simulink model "volo_agcdc_pipelined"  (R2012b)
settings: Solver=ode45  StartTime=0.0  StopTime=1000  RelTol=1e-3
PreLoadFcn:
  | volo_agcdc_init
InitFcn:
  | volo_agcdc_init
StartFcn:
  | volo_agcdc_init
values from neighbouring files (symbols this model uses):
  agc_idleState = 0    [volo_agcdc_init.m]
  agc_numAddrBits = agc_numOutputs + agc_numStateBits    [volo_agcdc_init.m]
  regDCRemoval_AvgLength = 64    [volo_agcdc_init.m]
  regSatDet_NumSamples = 16    [volo_agcdc_init.m]
undefined symbols (not defined in the file or in its folder): gcbh, xlBlockLoadCallback, xlGetNormalizedPeriod
libraries: xbsIndex_r4 x681, xbsEDKLib_r4 x1
(part 6 of 7)

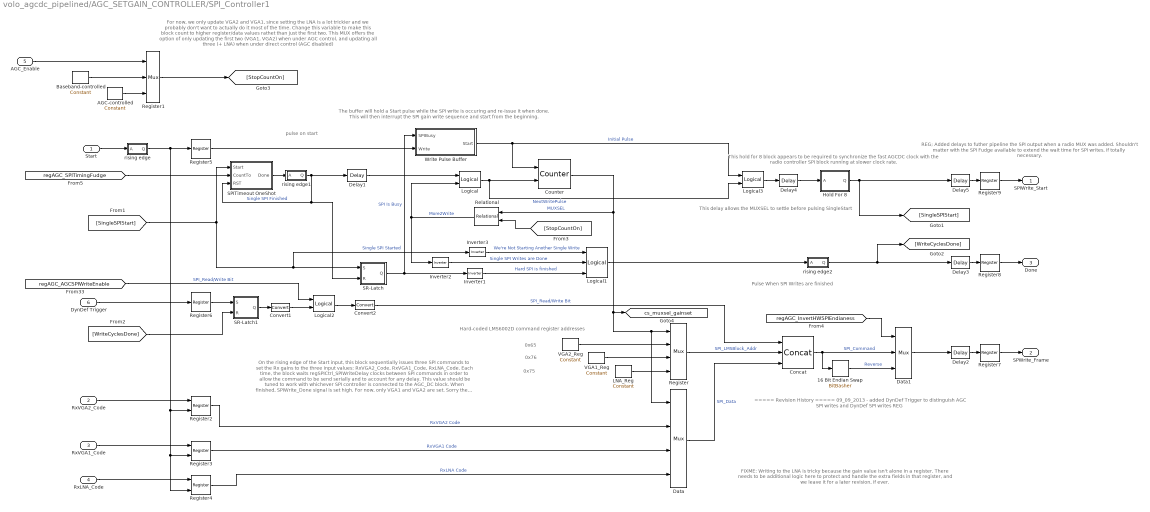
== system volo_agcdc_pipelined/AGC_SETGAIN_CONTROLLER/SPI_Controller1 ==
  note: REG; Added delays to futher pipeline the SPI output when a radio MUX was added.
      | Shouldn't matter with the SPI Fudge available to extend the wait time for SPI writes,
      | if totally necessary.
  note: This hold for 8 block appears to be required
      | to synchronize the fast AGCDC clock with
      | the radio controller SPI block running at slower
      | clock rate.
  note: ===== Revision History =====
      | 09_09_2013 - added DynDef Trigger to distinguish AGC SPI writes and DynDef SPI writes REG
  note: FIXME: Writing to the LNA is tricky because the gain value isn't alone in a register. There needs
      | to be additional logic here to protect and handle the extra fields in that register, and we leave it
      | for a later revision, if ever.
  note: For now, we only update VGA2 and VGA1, since setting the LNA is a lot trickier and we
      | probably don't want to actually do it most of the time. Change this variable to make this
      | block count to higher register/data values rathet than just the first two. This MUX offers the
      | option of only updating the first two (VGA1, VGA2) when under AGC control, and updating all
      | three (+ LNA) when under direct control (AGC disabled)
  note: The buffer will hold a Start pulse while the SPI write is occuring and re-issue it when done.
      | This will then interrupt the SPI gain write sequence and start from the beginning.
  note: This delay allows the MUXSEL
      | to settle before pulsing SingleStart
  note: Pulse When SPI Writes are finished
  note: pulse on start
  note: 0x75
  note: 0x76
  note: 0x65
  note: Hard-coded LMS6002D command
      | register addresses
  note: On the rising edge of the Start input, this block sequentially issues three SPI commands
      | to set the Rx gains to the three input values: RxVGA2_Code, RxVGA1_Code, RxLNA_Code.
      | Each time, the block waits regSPICtrl_SPIWriteDelay clocks between SPI commands in order
      | to allow the command to be send serially and to account for any delay. This value should be tuned
      | to work with whichever SPI controller is connected to the AGC_DC block. When finished,
      | SPIWrite_Done signal is set high. For now, only VGA1 and VGA2 are set.
      | Sorry the logic is a cluster, that's my bad--we had some serious issues with the SPI controller block.
      | me@ryaneguerra.com
      | June 15, 2013
  Start : Inport
  RxVGA2_Code : Inport  Port=2
  RxVGA1_Code : Inport  Port=3
  RxLNA_Code : Inport  Port=4
  AGC_Enable : Inport  Port=5
  DynDef Trigger : Inport  Port=6
  16 Bit Endian Swap : xbsIndex_r4/BitBasher  bitexpr=|  display_expr=off  sr_1=1  arith_type1=Unsigned  bin_pt1=0  sr_2=2  arith_type2=Unsigned  bin_pt2=0  sr_3=3  arith_type3=Unsigned  bin_pt3=0  sr_4=4  arith_type4=Unsigned  bin_pt4=0  dbl_ovrd=off  block_type=bitbasher
      | <!DOCTYPE HTML PUBLIC "-//W3C//DTD HTML 4.0//EN" "http://www.w3.org/TR/REC-html40/strict.dtd">
      | <html><head><meta name="qrichtext" content="1" /><style type="text/css">
      | p, li { white-space: pre-wrap; }
      | </style></head><body style=" font-family:'MS Shell Dlg 2'; font-size:8.25pt; font-weight:400; font-style:normal;">
      | <p style=" margin-top:12px; margin-bottom:12px; margin-left:0px; margin-right:0px; -qt-block-indent:0; text-indent:0px;"><span style=" font-family:'MS Shell Dlg'; font-size:8pt;">a={b[0:15]}</span></p></body></html>
  AGC-controlled : xbsIndex_r4/Constant  const=1  gui_display_data_type=Fixed-point  arith_type=Unsigned  n_bits=2  bin_pt=0  preci_type=Single  exp_width=8  frac_width=24  explicit_period=off  period=1  equ=P=C  opselect=C  inp2=PCIN>>17  opr=+  inp1=P  carry=CIN  dbl_ovrd=off  block_type=constant
  Baseband-controlled : xbsIndex_r4/Constant  const=1  gui_display_data_type=Fixed-point  arith_type=Unsigned  n_bits=2  bin_pt=0  preci_type=Single  exp_width=8  frac_width=24  explicit_period=off  period=1  equ=P=C  opselect=C  inp2=PCIN>>17  opr=+  inp1=P  carry=CIN  dbl_ovrd=off  block_type=constant
  Concat : xbsIndex_r4/Concat  num_inputs=3  dbl_ovrd=off  block_type=concat
  Convert1 : xbsIndex_r4/Convert  gui_display_data_type=Boolean  arith_type=Boolean  n_bits=16  bin_pt=14  float_type=Single  exp_bits=8  fraction_bits=24  quantization=Truncate  overflow=Wrap  en=off  latency=0  dbl_ovrd=off  pipeline=off  block_type=convert
  Convert2 : xbsIndex_r4/Convert  gui_display_data_type=Fixed-point  arith_type=Unsigned  n_bits=1  bin_pt=0  float_type=Single  exp_bits=8  fraction_bits=24  quantization=Truncate  overflow=Wrap  en=off  latency=0  dbl_ovrd=off  pipeline=off  block_type=convert
  Counter : xbsIndex_r4/Counter  cnt_type=Free Running  cnt_to=Inf  operation=Up  start_count=0  cnt_by_val=1  arith_type=Unsigned  n_bits=2  bin_pt=0  load_pin=off  rst=on  en=on  explicit_period=on  period=1  dbl_ovrd=off  use_behavioral_HDL=off  implementation=Fabric  block_type=counter
  Data : xbsIndex_r4/Mux  inputs=3  en=off  latency=0  precision=Full  arith_type=Unsigned  n_bits=16  bin_pt=14  quantization=Truncate  overflow=Wrap  dbl_ovrd=off  block_type=mux
  Data1 : xbsIndex_r4/Mux  inputs=2  en=off  latency=0  precision=Full  arith_type=Unsigned  n_bits=16  bin_pt=14  quantization=Truncate  overflow=Wrap  dbl_ovrd=off  block_type=mux
  Delay{1..5} (5 alike) : xbsIndex_r4/Delay  rst=off  infoeditControl=Selection of Reset will increase slice count due to use of real FFs and instead of SRLs  en=off  latency=1  dbl_ovrd=off  reg_retiming=off  block_type=delay
  Hold For 8 : Subsystem
  Inverter1 : xbsIndex_r4/Inverter  en=off  latency=0  dbl_ovrd=off  block_type=inv
  Inverter2 : xbsIndex_r4/Inverter  en=off  latency=0  dbl_ovrd=off  block_type=inv
  Inverter3 : xbsIndex_r4/Inverter  en=off  latency=0  dbl_ovrd=off  block_type=inv
  LNA_Reg : xbsIndex_r4/Constant  const=hex2dec('75')  gui_display_data_type=Fixed-point  arith_type=Unsigned  n_bits=7  bin_pt=0  preci_type=Single  exp_width=8  frac_width=24  explicit_period=on  period=1  equ=P=C  opselect=C  inp2=PCIN>>17  opr=+  inp1=P  carry=CIN  dbl_ovrd=off  block_type=constant
  Logical : xbsIndex_r4/Logical  logical_function=AND  inputs=2  en=off  latency=0  precision=Full  arith_type=Unsigned  n_bits=16  bin_pt=0  align_bp=on  dbl_ovrd=off  block_type=logical
  Logical1 : xbsIndex_r4/Logical  logical_function=AND  inputs=3  en=off  latency=0  precision=Full  arith_type=Unsigned  n_bits=16  bin_pt=0  align_bp=on  dbl_ovrd=off  block_type=logical
  Logical2 : xbsIndex_r4/Logical  logical_function=OR  inputs=2  en=off  latency=0  precision=Full  arith_type=Unsigned  n_bits=16  bin_pt=0  align_bp=on  dbl_ovrd=off  block_type=logical
  Logical3 : xbsIndex_r4/Logical  logical_function=OR  inputs=2  en=off  latency=0  precision=Full  arith_type=Unsigned  n_bits=16  bin_pt=0  align_bp=on  dbl_ovrd=off  block_type=logical
  Register : xbsIndex_r4/Mux  inputs=3  en=off  latency=0  precision=Full  arith_type=Unsigned  n_bits=16  bin_pt=14  quantization=Truncate  overflow=Wrap  dbl_ovrd=off  block_type=mux
  Register1 : xbsIndex_r4/Mux  inputs=2  en=off  latency=0  precision=Full  arith_type=Unsigned  n_bits=16  bin_pt=14  quantization=Truncate  overflow=Wrap  dbl_ovrd=off  block_type=mux
  Register2 : xbsIndex_r4/Register  init=0  rst=off  en=on  dbl_ovrd=off  block_type=register
  Register3 : xbsIndex_r4/Register  init=0  rst=off  en=on  dbl_ovrd=off  block_type=register
  Register4 : xbsIndex_r4/Register  init=0  rst=off  en=on  dbl_ovrd=off  block_type=register
  Register{5..9} (5 alike) : xbsIndex_r4/Register  init=0  rst=off  en=off  dbl_ovrd=off  block_type=register
  Relational : xbsIndex_r4/Relational  mode=a<b  en=off  latency=0  dbl_ovrd=off  block_type=relational
  SPITimeout OneShot : Subsystem
  SR-Latch : Subsystem
  SR-Latch1 : Subsystem
  VGA1_Reg : xbsIndex_r4/Constant  const=hex2dec('76')  gui_display_data_type=Fixed-point  arith_type=Unsigned  n_bits=7  bin_pt=0  preci_type=Single  exp_width=8  frac_width=24  explicit_period=on  period=1  equ=P=C  opselect=C  inp2=PCIN>>17  opr=+  inp1=P  carry=CIN  dbl_ovrd=off  block_type=constant
  VGA2_Reg : xbsIndex_r4/Constant  const=hex2dec('65')  gui_display_data_type=Fixed-point  arith_type=Unsigned  n_bits=7  bin_pt=0  preci_type=Single  exp_width=8  frac_width=24  explicit_period=on  period=1  equ=P=C  opselect=C  inp2=PCIN>>17  opr=+  inp1=P  carry=CIN  dbl_ovrd=off  block_type=constant
  Write Pulse Buffer : Subsystem
  rising edge : Subsystem
  rising edge1 : Subsystem
  rising edge2 : Subsystem
  SPIWrite_Start : Outport
  SPWrite_Frame : Outport  Port=2
  Done : Outport  Port=3
  tag scope: cs_muxsel_gainset=global
  wires:
  Register3/1 -> Data/3  "RxVGA1 Code"
  Register4/1 -> Data/4  "RxLNA Code"
  Register2/1 -> Data/2  "RxVGA2 Code"
  VGA1_Reg/1 -> Register/3
  LNA_Reg/1 -> Register/4
  VGA2_Reg/1 -> Register/2
  Data/1 -> Concat/3  "SPI_Data"
  Register/1 -> Concat/2  "SPI_LMSBlock_Addr"
  Concat/1 -> Data1/2, 16 Bit Endian Swap/1  "SPI_Command"
  Counter/1 -> Data/1, Register/1, [cs_muxsel_gainset], Relational/1  "MUXSEL"
  [StopCountOn] -> Relational/2
  Logical1/1 -> rising edge2/1(A)
  Register1/1 -> [StopCountOn]
  Logical2/1 -> Convert2/1
  SR-Latch/1(Q) -> Inverter1/1, Write Pulse Buffer/1(SPIBusy)  "SPI Is Busy"
  Relational/1 -> Inverter2/1, Logical/2  "More2Write"
  rising edge1/1(Q) -> SPITimeout OneShot/3(RST), SR-Latch/2(R), Delay1/1  "Single SPI Finished"
  Inverter2/1 -> Logical1/2  "Single SPI Writes are Done"
  Start/1 -> rising edge/1(A)
  Register5/1 -> Write Pulse Buffer/2(Write)
  Write Pulse Buffer/1(Start) -> Logical3/1, Counter/1  "Initial Pulse"
  rising edge2/1(Q) -> Delay3/1, [WriteCyclesDone]
  [SingleSPIStart] -> SR-Latch/1(S), Inverter3/1, SPITimeout OneShot/1(Start)  "Single SPI Started"
  Inverter1/1 -> Logical1/3  "Hard SPI is finished"
  [regAGC_SPITimingFudge] -> SPITimeout OneShot/2(CountTo)
  SPITimeout OneShot/1(Done) -> rising edge1/1(A)
  Delay1/1 -> Logical/1
  Logical/1 -> Logical3/2, Counter/2  "NextWritePulse"
  Inverter3/1 -> Logical1/1  "We're Not Starting Another Single Write"
  AGC-controlled/1 -> Register1/3
  Baseband-controlled/1 -> Register1/2
  AGC_Enable/1 -> Register1/1
  [regAGC_AGCSPIWriteEnable] -> Logical2/1  "SPI_Read/Write Bit"
  DynDef Trigger/1 -> Register6/1
  SR-Latch1/1(Q) -> Convert1/1
  [WriteCyclesDone] -> SR-Latch1/2(R)
  Convert1/1 -> Logical2/2
  Convert2/1 -> Concat/1  "SPI_Read/Write Bit"
  [regAGC_InvertHWSPIEndianess] -> Data1/1
  16 Bit Endian Swap/1 -> Data1/3  "Reverse"
  Data1/1 -> Delay2/1
  RxLNA_Code/1 -> Register4/1
  RxVGA1_Code/1 -> Register3/1
  RxVGA2_Code/1 -> Register2/1
  rising edge/1(Q) -> Register4/2, Register3/2, Register2/2, Register5/1
  Register6/1 -> SR-Latch1/1(S)
  Hold For 8/1(Q) -> Delay5/1, [SingleSPIStart]
  Logical3/1 -> Delay4/1
  Delay4/1 -> Hold For 8/1(A)
  Register7/1 -> SPWrite_Frame/1
  Delay2/1 -> Register7/1
  Delay3/1 -> Register8/1
  Register8/1 -> Done/1
  Register9/1 -> SPIWrite_Start/1
  Delay5/1 -> Register9/1

== system volo_agcdc_pipelined/AGC_SETGAIN_CONTROLLER/SR-Latch ==
  S : Inport
  R : Inport  Port=2
  Register : xbsIndex_r4/Register  init=0  rst=on  en=on  dbl_ovrd=off  block_type=register
  Q : Outport
  wires:
  S/1 -> Register/3, Register/1
  Register/1 -> Q/1
  R/1 -> Register/2

== system volo_agcdc_pipelined/AGC_SETGAIN_CONTROLLER/rising edge ==
  note: rising edge
  A : Inport
  Delay1 : xbsIndex_r4/Delay  rst=off  infoeditControl=Selection of Reset will increase slice count due to use of real FFs and instead of SRLs  en=off  latency=1  dbl_ovrd=off  reg_retiming=off  block_type=delay
  Inverter2 : xbsIndex_r4/Inverter  en=off  latency=0  dbl_ovrd=off  block_type=inv
  Logical2 : xbsIndex_r4/Logical  logical_function=AND  inputs=2  en=off  latency=0  precision=Full  arith_type=Unsigned  n_bits=16  bin_pt=0  align_bp=on  dbl_ovrd=off  block_type=logical
  Q : Outport
  wires:
  Logical2/1 -> Q/1
  A/1 -> Logical2/1, Delay1/1
  Delay1/1 -> Inverter2/1
  Inverter2/1 -> Logical2/2

== system volo_agcdc_pipelined/DC_REMOVAL/Sliding Sum 64_1 ==
  in : Inport
  rst : Inport  Port=2
  RxValid : Inport  Port=3
  Accum1 : xbsIndex_r4/Accumulator  operation=Add  n_bits=22  overflow=Saturate  scale=1  rst=on  infoeditControl=reset for floating point data type must be asserted for a minimum of 2 cycles  hasbypass=off  en=on  latency=0  dbl_ovrd=off  msb_inp=100  msb=100  lsb=-100  use_behavioral_HDL=on  implementation=Fabric  block_type=accum
      settings: xl_area=[12 23 0 22 0 0 0]  block_version=VER_STRING_GOES_HERE
  AddSub1 : xbsIndex_r4/AddSub  mode=Subtraction  use_carryin=off  use_carryout=off  en=off  latency=0  precision=Full  arith_type="Signed  (2's comp)"  n_bits=36  bin_pt=28  quantization=Truncate  overflow=Saturate  dbl_ovrd=off  use_behavioral_HDL=on  hw_selection=Fabric  pipelined=off  use_rpm=off  block_type=addsub
      settings: xl_area=[9 18 0 17 0 0 0]  block_version=VER_STRING_GOES_HERE
  Delay : xbsIndex_r4/Delay  rst=on  infoeditControl=Selection of Reset will increase slice count due to use of real FFs and instead of SRLs  en=on  latency=64  dbl_ovrd=off  reg_retiming=off  block_type=delay
  Out : Outport
  wires:
  Accum1/1 -> Out/1  "Sum"
  in/1 -> Delay/1, AddSub1/1  "Instantaneous"
  AddSub1/1 -> Accum1/1
  rst/1 -> Delay/2, Accum1/2
  Delay/1 -> AddSub1/2
  RxValid/1 -> Accum1/3, Delay/3

== system volo_agcdc_pipelined/DC_REMOVAL/Sliding Sum 64_2 ==
  in : Inport
  rst : Inport  Port=2
  RxValid : Inport  Port=3
  Accum1 : xbsIndex_r4/Accumulator  operation=Add  n_bits=22  overflow=Saturate  scale=1  rst=on  infoeditControl=reset for floating point data type must be asserted for a minimum of 2 cycles  hasbypass=off  en=on  latency=0  dbl_ovrd=off  msb_inp=100  msb=100  lsb=-100  use_behavioral_HDL=on  implementation=Fabric  block_type=accum
      settings: xl_area=[12 23 0 22 0 0 0]  block_version=VER_STRING_GOES_HERE
  AddSub1 : xbsIndex_r4/AddSub  mode=Subtraction  use_carryin=off  use_carryout=off  en=off  latency=0  precision=Full  arith_type="Signed  (2's comp)"  n_bits=36  bin_pt=28  quantization=Truncate  overflow=Saturate  dbl_ovrd=off  use_behavioral_HDL=on  hw_selection=Fabric  pipelined=off  use_rpm=off  block_type=addsub
      settings: xl_area=[9 18 0 17 0 0 0]  block_version=VER_STRING_GOES_HERE
  Delay : xbsIndex_r4/Delay  rst=on  infoeditControl=Selection of Reset will increase slice count due to use of real FFs and instead of SRLs  en=on  latency=64  dbl_ovrd=off  reg_retiming=off  block_type=delay
  Out : Outport
  wires:
  Accum1/1 -> Out/1  "Sum"
  in/1 -> Delay/1, AddSub1/1  "Instantaneous"
  AddSub1/1 -> Accum1/1
  rst/1 -> Delay/2, Accum1/2
  Delay/1 -> AddSub1/2
  RxValid/1 -> Delay/3, Accum1/3

== system volo_agcdc_pipelined/DC_REMOVAL/Valid Avg Counter ==
  RxValid : Inport
  RST : Inport  Port=2
  Constant : xbsIndex_r4/Constant  const=64  gui_display_data_type=Fixed-point  arith_type=Unsigned  n_bits=7  bin_pt=0  preci_type=Single  exp_width=8  frac_width=24  explicit_period=on  period=1  equ=P=C  opselect=C  inp2=PCIN>>17  opr=+  inp1=P  carry=CIN  dbl_ovrd=off  block_type=constant
  Counter : xbsIndex_r4/Counter  cnt_type=Free Running  cnt_to=10  operation=Up  start_count=0  cnt_by_val=1  arith_type=Unsigned  n_bits=ceil(log(regDCRemoval_AvgLength)/log(2))+1  bin_pt=0  load_pin=off  rst=on  en=on  explicit_period=on  period=1  dbl_ovrd=off  use_behavioral_HDL=off  implementation=Fabric  block_type=counter
  Inverter : xbsIndex_r4/Inverter  en=off  latency=0  dbl_ovrd=off  block_type=inv
  Logical : xbsIndex_r4/Logical  logical_function=AND  inputs=2  en=off  latency=0  precision=Full  arith_type=Unsigned  n_bits=16  bin_pt=0  align_bp=on  dbl_ovrd=off  block_type=logical
  Relational4 : xbsIndex_r4/Relational  mode=a>b  en=off  latency=0  dbl_ovrd=off  block_type=relational
  DCMeas_Good : Outport
  wires:
  RxValid/1 -> Logical/1
  RST/1 -> Counter/1
  Relational4/1 -> DCMeas_Good/1, Inverter/1  "DCMeasure_Good"
  Counter/1 -> Relational4/1
  Constant/1 -> Relational4/2
  Inverter/1 -> Logical/2  "keep_counting"
  Logical/1 -> Counter/2

== system volo_agcdc_pipelined/DynamicNoiseFloorAdjustment/Bounds Checking ==
  note: Note, it is not expected that the input is both above the max and below the min;
      | this is undefined behavior. Just to make sure nothing stupid happened, we'll put the
      | gain at MAX if that happens.
  note: Checks for rational bounds on the Dyn Default Gain,
      | otherwise, the output value is the rail value.
  NextGain_In : Inport
  Concat : xbsIndex_r4/Concat  num_inputs=2  dbl_ovrd=off  block_type=concat
  Delay1 : xbsIndex_r4/Delay  rst=off  infoeditControl=Selection of Reset will increase slice count due to use of real FFs and instead of SRLs  en=off  latency=1  dbl_ovrd=off  reg_retiming=off  block_type=delay
  Delay5 : xbsIndex_r4/Delay  rst=off  infoeditControl=Selection of Reset will increase slice count due to use of real FFs and instead of SRLs  en=off  latency=1  dbl_ovrd=off  reg_retiming=off  block_type=delay
  Mux : xbsIndex_r4/Mux  inputs=4  en=off  latency=0  precision=Full  arith_type=Unsigned  n_bits=16  bin_pt=14  quantization=Truncate  overflow=Wrap  dbl_ovrd=off  block_type=mux
  Relational : xbsIndex_r4/Relational  mode=a>b  en=off  latency=0  dbl_ovrd=off  block_type=relational
  Relational1 : xbsIndex_r4/Relational  mode=a<b  en=off  latency=0  dbl_ovrd=off  block_type=relational
  NextGain_Out : Outport
  wires:
  [regAGC_DynAdjustment_MinDefaultGain] -> Mux/4, Relational1/2  "Min Default Gain"
  [regAGC_DynAdjustment_MaxDefaultGain] -> Mux/5, Mux/3, Relational/2  "Max Default Gain"
  NextGain_In/1 -> Relational1/1, Relational/1, Delay1/1  "NExt Gain"
  Relational1/1 -> Concat/1  "IN < MIN"
  Relational/1 -> Concat/2  "IN > MAX"
  Concat/1 -> Delay5/1
  Delay5/1 -> Mux/1
  Delay1/1 -> Mux/2  "Next Gain"
  Mux/1 -> NextGain_Out/1

== system volo_agcdc_pipelined/DynamicNoiseFloorAdjustment/Default Gain Change Holdoff Timer ==
  Current_Default : Inport
  Next_Default : Inport  Port=2
  RST : Inport  Port=3
  Always Update : xbsIndex_r4/Constant  const=1  gui_display_data_type=Boolean  arith_type=Boolean  n_bits=3  bin_pt=0  preci_type=Single  exp_width=8  frac_width=24  explicit_period=off  period=1  equ=P=C  opselect=C  inp2=PCIN>>17  opr=+  inp1=P  carry=CIN  dbl_ovrd=off  block_type=constant
  Logical3 : xbsIndex_r4/Logical  logical_function=OR  inputs=2  en=off  latency=0  precision=Full  arith_type=Unsigned  n_bits=16  bin_pt=0  align_bp=on  dbl_ovrd=off  block_type=logical
  LongCorrTimeout_OneShot : Subsystem
  Mux1 : xbsIndex_r4/Mux  inputs=2  en=off  latency=0  precision=Full  arith_type=Unsigned  n_bits=16  bin_pt=14  quantization=Truncate  overflow=Wrap  dbl_ovrd=off  block_type=mux
  Mux3 : xbsIndex_r4/Mux  inputs=2  en=off  latency=0  precision=Full  arith_type=Unsigned  n_bits=16  bin_pt=14  quantization=Truncate  overflow=Wrap  dbl_ovrd=off  block_type=mux
  Relational2 : xbsIndex_r4/Relational  mode=a!=b  en=off  latency=0  dbl_ovrd=off  block_type=relational
  Timer Never Counts : xbsIndex_r4/Constant  const=0  gui_display_data_type=Boolean  arith_type=Boolean  n_bits=3  bin_pt=0  preci_type=Single  exp_width=8  frac_width=24  explicit_period=off  period=1  equ=P=C  opselect=C  inp2=PCIN>>17  opr=+  inp1=P  carry=CIN  dbl_ovrd=off  block_type=constant
  rising edge1 : Subsystem
  UpdateDefault : Outport
  IsCounting : Outport  Port=2
  wires:
  [regAGC_DynAdjustment_HoldoffTimer] -> LongCorrTimeout_OneShot/2(CountTo)
  LongCorrTimeout_OneShot/1(Done) -> rising edge1/1(A)
  RST/1 -> Logical3/1  "A good payload (maybe good packet) was received; halt any pending changes"
  rising edge1/1(Q) -> Logical3/2, Mux3/3
  Logical3/1 -> LongCorrTimeout_OneShot/3(RST)
  Always Update/1 -> Mux3/2
  [regAGC_DynAdjustment_EnHoldoffTimer] -> Mux1/1, Mux3/1  "Enable Holdoff Timer"
  Mux3/1 -> UpdateDefault/1
  Relational2/1 -> LongCorrTimeout_OneShot/1(Start)  "Default Needs Update"
  Current_Default/1 -> Relational2/1
  Next_Default/1 -> Relational2/2
  Timer Never Counts/1 -> Mux1/2
  Mux1/1 -> IsCounting/1
  LongCorrTimeout_OneShot/2(IsCounting) -> Mux1/3

== system volo_agcdc_pipelined/DynamicNoiseFloorAdjustment/rising edge2 ==
  note: rising edge
  A : Inport
  Convert : xbsIndex_r4/Convert  gui_display_data_type=Boolean  arith_type=Boolean  n_bits=16  bin_pt=14  float_type=Single  exp_bits=8  fraction_bits=24  quantization=Truncate  overflow=Wrap  en=off  latency=0  dbl_ovrd=off  pipeline=off  block_type=convert
  Delay1 : xbsIndex_r4/Delay  rst=off  infoeditControl=Selection of Reset will increase slice count due to use of real FFs and instead of SRLs  en=off  latency=1  dbl_ovrd=off  reg_retiming=off  block_type=delay
  Inverter2 : xbsIndex_r4/Inverter  en=off  latency=0  dbl_ovrd=off  block_type=inv
  Logical2 : xbsIndex_r4/Logical  logical_function=AND  inputs=2  en=off  latency=0  precision=Full  arith_type=Unsigned  n_bits=16  bin_pt=0  align_bp=on  dbl_ovrd=off  block_type=logical
  Q : Outport
  wires:
  Convert/1 -> Q/1
  Inverter2/1 -> Logical2/2
  Delay1/1 -> Inverter2/1
  A/1 -> Delay1/1, Logical2/1
  Logical2/1 -> Convert/1

== system volo_agcdc_pipelined/Ext_PktDet_Delay/Ext Pkt Det Delay  ==
  note: Note: If the input value changes at any time while the oneshot is
      | counting, it will be reset and Out will never change state
  In : Inport
  32Bit_OneShot : Subsystem
  Inverter : xbsIndex_r4/Inverter  en=off  latency=0  dbl_ovrd=off  block_type=inv
  Inverter1 : xbsIndex_r4/Inverter  en=off  latency=0  dbl_ovrd=off  block_type=inv
  Logical : xbsIndex_r4/Logical  logical_function=XOR  inputs=2  en=off  latency=0  precision=Full  arith_type=Unsigned  n_bits=16  bin_pt=0  align_bp=on  dbl_ovrd=off  block_type=logical
  Logical1 : xbsIndex_r4/Logical  logical_function=OR  inputs=2  en=off  latency=0  precision=Full  arith_type=Unsigned  n_bits=16  bin_pt=0  align_bp=on  dbl_ovrd=off  block_type=logical
  Old Configurable Delay Block : Subsystem  Commented=on
  Register : xbsIndex_r4/Register  init=0  rst=off  en=on  dbl_ovrd=off  block_type=register
  rising edge : Subsystem
  Out : Outport
  wires:
  In/1 -> Inverter1/1, Register/1, Logical/2  "input"
  Logical/1 -> 32Bit_OneShot/1(Start), Inverter/1  "output unsynched"
  [regWSD_ExtPktDetectDelayCount] -> 32Bit_OneShot/2(CountTo)
  32Bit_OneShot/1(Done) -> rising edge/1(A)
  Inverter/1 -> 32Bit_OneShot/3(RST)  "output synched"
  rising edge/1(Q) -> Logical1/1
  Register/1 -> Logical/1, Out/1  "output"
  Logical1/1 -> Register/2
  Inverter1/1 -> Logical1/2

== system volo_agcdc_pipelined/Ext_PktDet_Delay/S-R Latch2 ==
  S : Inport
  R : Inport  Port=2
  Constant1 : xbsIndex_r4/Constant  const=1  gui_display_data_type=Fixed-point  arith_type=Boolean  n_bits=1  bin_pt=0  preci_type=Single  exp_width=8  frac_width=24  explicit_period=off  period=1  equ=P=C  opselect=C  inp2=PCIN>>17  opr=+  inp1=P  carry=CIN  dbl_ovrd=off  block_type=constant
      settings: block_version=VER_STRING_GOES_HERE
  Convert : xbsIndex_r4/Convert  gui_display_data_type=Fixed-point  arith_type=Boolean  n_bits=16  bin_pt=14  float_type=Single  exp_bits=8  fraction_bits=24  quantization=Truncate  overflow=Wrap  en=off  latency=0  dbl_ovrd=off  pipeline=off  block_type=convert
      settings: block_version=10.1.3
  Convert1 : xbsIndex_r4/Convert  gui_display_data_type=Fixed-point  arith_type=Boolean  n_bits=16  bin_pt=14  float_type=Single  exp_bits=8  fraction_bits=24  quantization=Truncate  overflow=Wrap  en=off  latency=0  dbl_ovrd=off  pipeline=off  block_type=convert
      settings: block_version=10.1.3
  Register2 : xbsIndex_r4/Register  init=0  rst=on  en=on  dbl_ovrd=off  block_type=register
      settings: xl_area=[1 1 0 0 0 0 0]  block_version=VER_STRING_GOES_HERE
  Q : Outport
  wires:
  Convert1/1 -> Register2/3
  Convert/1 -> Register2/2
  S/1 -> Convert1/1
  Register2/1 -> Q/1
  R/1 -> Convert/1
  Constant1/1 -> Register2/1

== system volo_agcdc_pipelined/MEASURE_AVGPWR/Magnitude Squared - Delay 2 ==
  note: Ryan: FIXME - i effed with this
  I : Inport
  Q : Inport  Port=2
  AddSub1 : xbsIndex_r4/AddSub  mode=Addition  use_carryin=off  use_carryout=off  en=off  latency=1  precision=Full  arith_type=Unsigned  n_bits=16  bin_pt=15  quantization=Truncate  overflow=Saturate  dbl_ovrd=off  use_behavioral_HDL=on  hw_selection=Fabric  pipelined=off  use_rpm=on  block_type=addsub
      settings: xl_area=[12 22 0 22 0 0 0]  block_version=VER_STRING_GOES_HERE
  Gateway Out{,1..5} (6 alike) : xbsIndex_r4/Gateway Out  inherit_from_input=off  hdl_port=off  timing_constraint=None  locs_specified=off  LOCs={}  UseAsDAC=off  DACChannel='1'  block_type=gatewayout
  Mult1 : xbsIndex_r4/Mult  precision=Full  arith_type=Unsigned  n_bits=16  bin_pt=16  quantization=Truncate  overflow=Saturate  en=off  latency=1  dbl_ovrd=off  use_behavioral_HDL=off  opt=Speed  use_embedded=on  optimum_pipeline=off  pipeline=on  use_rpm=off  placement_style=Rectangular shape  block_type=mult
      settings: xl_area=[63 105 0 106 0 4 0]  block_version=VER_STRING_GOES_HERE
  Mult4 : xbsIndex_r4/Mult  precision=Full  arith_type=Unsigned  n_bits=16  bin_pt=16  quantization=Truncate  overflow=Saturate  en=off  latency=1  dbl_ovrd=off  use_behavioral_HDL=off  opt=Speed  use_embedded=on  optimum_pipeline=off  pipeline=on  use_rpm=off  placement_style=Rectangular shape  block_type=mult
      settings: xl_area=[63 105 0 106 0 4 0]  block_version=VER_STRING_GOES_HERE
  Scope : Scope  NumInputPorts=6
      settings: ShowLegends=on  YMin=-5~-5~-5~-5~-5~-5  YMax=5~5~5~5~5~5  SaveName=ScopeData5
  Mag : Outport
  wires:
  AddSub1/1 -> Mag/1
  Mult1/1 -> Gateway Out3/1, AddSub1/2
  Mult4/1 -> Gateway Out2/1, AddSub1/1
  Gateway Out/1 -> Scope/1
  Gateway Out1/1 -> Scope/2
  Gateway Out2/1 -> Scope/3
  Gateway Out3/1 -> Scope/4
  I/1 -> Gateway Out4/1, Mult4/2, Mult4/1, Gateway Out/1
  Q/1 -> Gateway Out5/1, Mult1/1, Mult1/2, Gateway Out1/1
  Gateway Out4/1 -> Scope/5
  Gateway Out5/1 -> Scope/6

== system volo_agcdc_pipelined/MEASURE_AVGPWR/len-32 Sliding Sum, dly 2 ==
  note: This block must be held in reset long enough so that LEN samples have passed.
      | This will flush the ASR of any non-zero samples and let the averager block reset.
  In : Inport
  rst : Inport  Port=2
  RxValid : Inport  Port=3
  Accum1 : xbsIndex_r4/Accumulator  operation=Add  n_bits=32  overflow=Saturate  scale=1  rst=on  infoeditControl=reset for floating point data type must be asserted for a minimum of 2 cycles  hasbypass=off  en=on  latency=0  dbl_ovrd=off  msb_inp=100  msb=100  lsb=-100  use_behavioral_HDL=on  implementation=Fabric  block_type=accum
      settings: xl_area=[12 23 0 22 0 0 0]  block_version=VER_STRING_GOES_HERE
  AddSub1 : xbsIndex_r4/AddSub  mode=Subtraction  use_carryin=off  use_carryout=off  en=off  latency=0  precision=Full  arith_type="Signed  (2's comp)"  n_bits=36  bin_pt=28  quantization=Truncate  overflow=Saturate  dbl_ovrd=off  use_behavioral_HDL=on  hw_selection=Fabric  pipelined=off  use_rpm=off  block_type=addsub
      settings: xl_area=[9 18 0 17 0 0 0]  block_version=VER_STRING_GOES_HERE
  Constant : xbsIndex_r4/Constant  const=0  gui_display_data_type=Fixed-point  arith_type=Signed (2's comp)  n_bits=16  bin_pt=14  preci_type=Single  exp_width=8  frac_width=24  explicit_period=off  period=1  equ=P=C  opselect=C  inp2=PCIN>>17  opr=+  inp1=P  carry=CIN  dbl_ovrd=off  block_type=constant
  Delay{1..3,5} (4 alike) : xbsIndex_r4/Delay  rst=off  infoeditControl=Selection of Reset will increase slice count due to use of real FFs and instead of SRLs  en=off  latency=1  dbl_ovrd=off  reg_retiming=off  block_type=delay
  Delay4 : xbsIndex_r4/Delay  rst=off  infoeditControl=Selection of Reset will increase slice count due to use of real FFs and instead of SRLs  en=on  latency=32  dbl_ovrd=off  reg_retiming=off  block_type=delay
  Mux : xbsIndex_r4/Mux  inputs=2  en=off  latency=0  precision=Full  arith_type=Unsigned  n_bits=16  bin_pt=14  quantization=Truncate  overflow=Wrap  dbl_ovrd=off  block_type=mux
  Out : Outport
  wires:
  Delay4/1 -> AddSub1/2
  AddSub1/1 -> Delay3/1
  Mux/1 -> Delay4/1, AddSub1/1  "Instantaneous"
  Accum1/1 -> Delay5/1  "Sum Power"
  rst/1 -> Mux/1, Delay1/1  "Reset"
  In/1 -> Mux/2  "Instantaneous"
  Constant/1 -> Mux/3
  RxValid/1 -> Delay4/2, Delay2/1
  Delay3/1 -> Accum1/1
  Delay1/1 -> Accum1/2
  Delay2/1 -> Accum1/3
  Delay5/1 -> Out/1

== system volo_agcdc_pipelined/PACKET_DETECTION/Auto-Corr Pkt Det ==
  note: pipeline delay
  note: Note: I added this MUX here to experiment with different
      | ways of detecting the packet, as well as allowing flexibility
      | for different designs that may use this pCore. REG
  RST : Inport
  Rx_Valid : Inport  Port=2
  DCR_I : Inport  Port=3
  DCR_Q : Inport  Port=4
  Filt_I : Inport  Port=5
  Filt_Q : Inport  Port=6
  Auto Corr : Subsystem
  Auto Corr Pkt Det : Scope  NumInputPorts=7
      settings: TimeRange=10000  YMin=-0.15~-0.2~0~0~-1~-1~-1  YMax=0.15~0.2~0.07~0.07~1~1~1  SaveName=ScopeData28
  Decision : Subsystem
  Delay5 : xbsIndex_r4/Delay  rst=off  infoeditControl=Selection of Reset will increase slice count due to use of real FFs and instead of SRLs  en=off  latency=1  dbl_ovrd=off  reg_retiming=off  block_type=delay
  Mag : Subsystem
  Mux : xbsIndex_r4/Mux  inputs=2  en=off  latency=0  precision=Full  arith_type=Unsigned  n_bits=16  bin_pt=14  quantization=Truncate  overflow=Wrap  dbl_ovrd=off  block_type=mux
  Mux1 : xbsIndex_r4/Mux  inputs=2  en=off  latency=0  precision=Full  arith_type=Unsigned  n_bits=16  bin_pt=14  quantization=Truncate  overflow=Wrap  dbl_ovrd=off  block_type=mux
  Register1 : xbsIndex_r4/Register  init=0  rst=off  en=off  dbl_ovrd=off  block_type=register
  Register2 : xbsIndex_r4/Register  init=0  rst=off  en=off  dbl_ovrd=off  block_type=register
  Register3 : xbsIndex_r4/Register  init=0  rst=off  en=off  dbl_ovrd=off  block_type=register
  done{1..6} (6 alike) : xbsIndex_r4/Gateway Out  inherit_from_input=off  hdl_port=off  timing_constraint=None  locs_specified=off  LOCs={}  UseAsDAC=off  DACChannel='1'  block_type=gatewayout
      settings: infoedit="Gateway out block.  Converts Xilinx fixed point inputs into ouputs of type Simulink integer, double, or fixed point.<P><P>Hardware notes:  In hardware these blocks become top level output ports or are discarded, depending on how they are configured."  xl_area=[0 0 0 0 1 0 0]  block_version=VER_STRING_GOES_HERE
  PktDet : Outport
  wires:
  done4/1 -> Auto Corr Pkt Det/1
  done2/1 -> Auto Corr Pkt Det/2
  done6/1 -> Auto Corr Pkt Det/5
  Register1/1 -> Auto Corr/2(I), Mag/2(I), done4/1  "Registered_I"
  Register3/1 -> Auto Corr/3(Q), Mag/3(Q), done2/1  "Registered_Q"
  Register2/1 -> Auto Corr/1(Valid), Mag/1(Valid)  "Registered_Valid"
  Auto Corr/1(Corr) -> Decision/2(Corr), done5/1
  Mag/1(Mag Sq) -> Decision/3(Mag), done3/1
  RST/1 -> Decision/1(PktDet Reset), done1/1
  done5/1 -> Auto Corr Pkt Det/3
  done3/1 -> Auto Corr Pkt Det/4
  Decision/1(PktDet) -> done6/1, Delay5/1
  done1/1 -> Auto Corr Pkt Det/6
  [regAGC_AutoCorrInSel] -> Mux1/1, Mux/1
  Filt_I/1 -> Mux/3
  Filt_Q/1 -> Mux1/3
  Rx_Valid/1 -> Register2/1
  Mux/1 -> Register1/1
  Mux1/1 -> Register3/1
  Delay5/1 -> PktDet/1
  DCR_I/1 -> Mux/2
  DCR_Q/1 -> Mux1/2

== system volo_agcdc_pipelined/PACKET_DETECTION/CrossCorrelator Packet Detector (TODO) ==
  note: TODO
  RST : Inport
  DCR_I : Inport  Port=2
  DCR_Q : Inport  Port=3
  RxValid : Inport  Port=4
  Constant : xbsIndex_r4/Constant  const=0  gui_display_data_type=Boolean  arith_type=Boolean  n_bits=16  bin_pt=14  preci_type=Single  exp_width=8  frac_width=24  explicit_period=off  period=1  equ=P=C  opselect=C  inp2=PCIN>>17  opr=+  inp1=P  carry=CIN  dbl_ovrd=off  block_type=constant
  Terminator{,1..3} (4 alike) : Terminator
  PktDet : Outport
  wires:
  DCR_I/1 -> Terminator/1
  DCR_Q/1 -> Terminator1/1
  RST/1 -> Terminator2/1
  Constant/1 -> PktDet/1
  RxValid/1 -> Terminator3/1

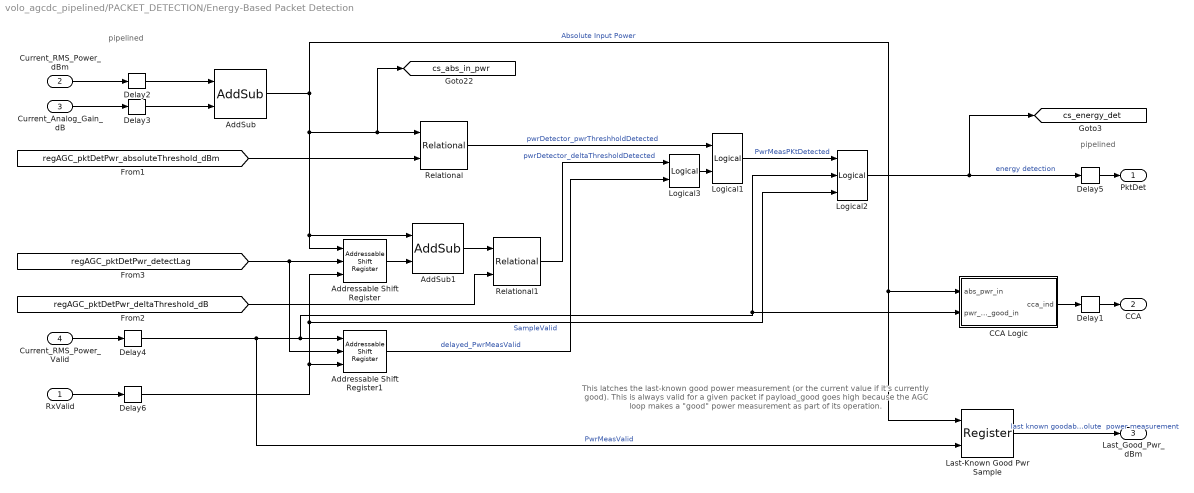
== system volo_agcdc_pipelined/PACKET_DETECTION/Energy-Based Packet Detection ==
  note: pipelined
  note: pipelined
  note: This latches the last-known good power measurement
      | (or the current value if it's currently good). This is always
      | valid for a given packet if payload_good goes high because
      | the AGC loop makes a "good" power measurement as part
      | of its operation.
  RxValid : Inport
  Current_RMS_Power_dBm : Inport  Port=2
  Current_Analog_Gain_dB : Inport  Port=3
  Current_RMS_Power_Valid : Inport  Port=4
  AddSub : xbsIndex_r4/AddSub  mode=Subtraction  use_carryin=off  use_carryout=off  en=off  latency=0  precision=Full  arith_type=Unsigned  n_bits=16  bin_pt=14  quantization=Truncate  overflow=Wrap  dbl_ovrd=off  use_behavioral_HDL=off  hw_selection=Fabric  pipelined=off  block_type=addsub
  AddSub1 : xbsIndex_r4/AddSub  mode=Subtraction  use_carryin=off  use_carryout=off  en=off  latency=0  precision=Full  arith_type=Unsigned  n_bits=16  bin_pt=14  quantization=Truncate  overflow=Wrap  dbl_ovrd=off  use_behavioral_HDL=off  hw_selection=Fabric  pipelined=off  block_type=addsub
  Addressable Shift Register : xbsIndex_r4/Addressable Shift Register  infer_latency=off  depth=64  initVector=[0]  en=on  dbl_ovrd=off  use_behavioral_HDL=off  Optimization=Resource  block_type=addrsr
      settings: infoedit="Delay of configurable length.  Any element in the delay line can be addressed and driven onto the output port.<br><br>Hardware notes: This block is implemented using SRL16s. If Virtex-4 or Spartan-3 device is used, multiple SRLC16s are cascaded together."
  Addressable Shift Register1 : xbsIndex_r4/Addressable Shift Register  infer_latency=off  depth=64  initVector=[0]  en=on  dbl_ovrd=off  use_behavioral_HDL=off  Optimization=Resource  block_type=addrsr
      settings: infoedit="Delay of configurable length.  Any element in the delay line can be addressed and driven onto the output port.<br><br>Hardware notes: This block is implemented using SRL16s. If Virtex-4 or Spartan-3 device is used, multiple SRLC16s are cascaded together."
  CCA Logic : Subsystem
  Delay{1..6} (6 alike) : xbsIndex_r4/Delay  rst=off  infoeditControl=Selection of Reset will increase slice count due to use of real FFs and instead of SRLs  en=off  latency=1  dbl_ovrd=off  reg_retiming=off  block_type=delay
  Last-Known Good Pwr Sample : xbsIndex_r4/Register  init=0  rst=off  en=on  dbl_ovrd=off  block_type=register
  Logical1 : xbsIndex_r4/Logical  logical_function=OR  inputs=2  en=off  latency=0  precision=Full  arith_type=Unsigned  n_bits=16  bin_pt=0  align_bp=on  dbl_ovrd=off  block_type=logical
  Logical2 : xbsIndex_r4/Logical  logical_function=AND  inputs=3  en=off  latency=0  precision=Full  arith_type=Unsigned  n_bits=16  bin_pt=0  align_bp=on  dbl_ovrd=off  block_type=logical
  Logical3 : xbsIndex_r4/Logical  logical_function=AND  inputs=2  en=off  latency=0  precision=Full  arith_type=Unsigned  n_bits=16  bin_pt=0  align_bp=on  dbl_ovrd=off  block_type=logical
  Relational : xbsIndex_r4/Relational  mode=a>b  en=off  latency=0  dbl_ovrd=off  block_type=relational
  Relational1 : xbsIndex_r4/Relational  mode=a>b  en=off  latency=0  dbl_ovrd=off  block_type=relational
  PktDet : Outport
  CCA : Outport  Port=2
  Last_Good_Pwr_dBm : Outport  Port=3
  tag scope: cs_abs_in_pwr=global, cs_energy_det=global
  wires:
  AddSub/1 -> Addressable Shift Register/1, AddSub1/1, [cs_abs_in_pwr], Relational/1, Last-Known Good Pwr Sample/1, CCA Logic/1(abs_pwr_in)  "Absolute Input Power"
  Addressable Shift Register1/1 -> Logical3/2  "delayed_PwrMeasValid"
  Current_RMS_Power_dBm/1 -> Delay2/1
  AddSub1/1 -> Relational1/1
  Logical1/1 -> Logical2/1  "PwrMeasPKtDetected"
  Logical3/1 -> Logical1/2
  Current_Analog_Gain_dB/1 -> Delay3/1
  [regAGC_pktDetPwr_deltaThreshold_dB] -> Relational1/2
  Relational1/1 -> Logical3/1  "pwrDetector_deltaThresholdDetected"
  Logical2/1 -> Delay5/1, [cs_energy_det]  "energy detection"
  Addressable Shift Register/1 -> AddSub1/2
  [regAGC_pktDetPwr_detectLag] -> Addressable Shift Register1/2, Addressable Shift Register/2
  [regAGC_pktDetPwr_absoluteThreshold_dBm] -> Relational/2
  Relational/1 -> Logical1/1  "pwrDetector_pwrThreshholdDetected"
  Last-Known Good Pwr Sample/1 -> Last_Good_Pwr_dBm/1  "last known goodabsolute  power measurement"
  Current_RMS_Power_Valid/1 -> Delay4/1
  RxValid/1 -> Delay6/1
  Delay2/1 -> AddSub/1
  Delay3/1 -> AddSub/2
  Delay4/1 -> Logical2/2, CCA Logic/2(pwr_measure_good_in), Addressable Shift Register1/1, Last-Known Good Pwr Sample/2  "PwrMeasValid"
  Delay6/1 -> Logical2/3, Addressable Shift Register/3, Addressable Shift Register1/3  "SampleValid"
  Delay5/1 -> PktDet/1
  CCA Logic/1(cca_ind) -> Delay1/1
  Delay1/1 -> CCA/1

== system volo_agcdc_pipelined/PACKET_DETECTION/anti-debouncer ==
  da_in : Inport
  rst : Inport  Port=2
  Delay{1..5} (5 alike) : xbsIndex_r4/Delay  rst=on  infoeditControl=Selection of Reset will increase slice count due to use of real FFs and instead of SRLs  en=off  latency=1  dbl_ovrd=off  reg_retiming=off  block_type=delay
  Logical6 : xbsIndex_r4/Logical  logical_function=OR  inputs=6  en=off  latency=0  precision=Full  arith_type=Unsigned  n_bits=16  bin_pt=0  align_bp=on  dbl_ovrd=off  block_type=logical
  da_ous : Outport
  wires:
  Delay3/1 -> Logical6/4, Delay4/1
  Delay4/1 -> Logical6/5, Delay5/1
  da_in/1 -> Delay1/1, Logical6/1
  Logical6/1 -> da_ous/1
  Delay1/1 -> Delay2/1, Logical6/2
  Delay2/1 -> Delay3/1, Logical6/3
  Delay5/1 -> Logical6/6
  rst/1 -> Delay2/2, Delay5/2, Delay4/2, Delay3/2, Delay1/2

== system volo_agcdc_pipelined/PACKET_DETECTION/rising edge ==
  note: rising edge
  A : Inport
  Delay1 : xbsIndex_r4/Delay  rst=off  infoeditControl=Selection of Reset will increase slice count due to use of real FFs and instead of SRLs  en=off  latency=1  dbl_ovrd=off  reg_retiming=off  block_type=delay
  Inverter2 : xbsIndex_r4/Inverter  en=off  latency=0  dbl_ovrd=off  block_type=inv
  Logical2 : xbsIndex_r4/Logical  logical_function=AND  inputs=2  en=off  latency=0  precision=Full  arith_type=Unsigned  n_bits=16  bin_pt=0  align_bp=on  dbl_ovrd=off  block_type=logical
  Q : Outport
  wires:
  Logical2/1 -> Q/1
  A/1 -> Logical2/1, Delay1/1
  Delay1/1 -> Inverter2/1
  Inverter2/1 -> Logical2/2

== system volo_agcdc_pipelined/SATURATION_DETECTOR/16-Sample Sliding Window Counter ==
  RxValid : Inport
  SatDet : Inport  Port=2
  RST : Inport  Port=3
  Accumulator1 : xbsIndex_r4/Accumulator  operation=Add  n_bits=ceil(log(regSatDet_NumSamples)/log(2)) + 2  overflow=Saturate  scale=1  rst=on  infoeditControl=reset for floating point data type must be asserted for a minimum of 2 cycles  hasbypass=off  en=on  latency=0  dbl_ovrd=off  msb_inp=100  msb=100  lsb=-100  use_behavioral_HDL=on  implementation=Fabric  block_type=accum
  AddSub1 : xbsIndex_r4/AddSub  mode=Subtraction  use_carryin=off  use_carryout=off  en=off  latency=0  precision=User Defined  arith_type="Signed  (2's comp)"  n_bits=2  bin_pt=0  quantization=Truncate  overflow=Saturate  dbl_ovrd=off  use_behavioral_HDL=off  hw_selection=Fabric  pipelined=off  block_type=addsub
  Convert1 : xbsIndex_r4/Convert  gui_display_data_type=Fixed-point  arith_type=Unsigned  n_bits=1  bin_pt=0  float_type=Single  exp_bits=8  fraction_bits=24  quantization=Truncate  overflow=Saturate  en=off  latency=0  dbl_ovrd=off  pipeline=off  block_type=convert
  Delay1 : xbsIndex_r4/Delay  rst=on  infoeditControl=Selection of Reset will increase slice count due to use of real FFs and instead of SRLs  en=on  latency=regSatDet_NumSamples  dbl_ovrd=off  reg_retiming=off  block_type=delay
  Sum : Outport
  wires:
  Delay1/1 -> AddSub1/2
  AddSub1/1 -> Accumulator1/1
  Accumulator1/1 -> Sum/1
  SatDet/1 -> Convert1/1
  Convert1/1 -> AddSub1/1, Delay1/1
  RST/1 -> Accumulator1/2, Delay1/2
  RxValid/1 -> Delay1/3, Accumulator1/3

== system volo_agcdc_pipelined/SATURATION_DETECTOR/16-Sample Sliding Window Counter1 ==
  RxValid : Inport
  SatDet : Inport  Port=2
  RST : Inport  Port=3
  Accumulator1 : xbsIndex_r4/Accumulator  operation=Add  n_bits=ceil(log(regSatDet_NumSamples)/log(2)) + 2  overflow=Saturate  scale=1  rst=on  infoeditControl=reset for floating point data type must be asserted for a minimum of 2 cycles  hasbypass=off  en=on  latency=0  dbl_ovrd=off  msb_inp=100  msb=100  lsb=-100  use_behavioral_HDL=on  implementation=Fabric  block_type=accum
  AddSub1 : xbsIndex_r4/AddSub  mode=Subtraction  use_carryin=off  use_carryout=off  en=off  latency=0  precision=User Defined  arith_type="Signed  (2's comp)"  n_bits=2  bin_pt=0  quantization=Truncate  overflow=Saturate  dbl_ovrd=off  use_behavioral_HDL=off  hw_selection=Fabric  pipelined=off  block_type=addsub
  Convert1 : xbsIndex_r4/Convert  gui_display_data_type=Fixed-point  arith_type=Unsigned  n_bits=1  bin_pt=0  float_type=Single  exp_bits=8  fraction_bits=24  quantization=Truncate  overflow=Saturate  en=off  latency=0  dbl_ovrd=off  pipeline=off  block_type=convert
  Delay1 : xbsIndex_r4/Delay  rst=on  infoeditControl=Selection of Reset will increase slice count due to use of real FFs and instead of SRLs  en=on  latency=regSatDet_NumSamples  dbl_ovrd=off  reg_retiming=off  block_type=delay
  Sum : Outport
  wires:
  Delay1/1 -> AddSub1/2
  AddSub1/1 -> Accumulator1/1
  Accumulator1/1 -> Sum/1
  SatDet/1 -> Convert1/1
  Convert1/1 -> AddSub1/1, Delay1/1
  RST/1 -> Accumulator1/2, Delay1/2
  RxValid/1 -> Delay1/3, Accumulator1/3

== system volo_agcdc_pipelined/TOP_LEVEL_AGC_TIMING/HoldUntilReset2 ==
  A : Inport
  RST : Inport  Port=2
  Register : xbsIndex_r4/Register  init=0  rst=on  en=on  dbl_ovrd=off  block_type=register
  Q : Outport
  wires:
  A/1 -> Register/3, Register/1
  Register/1 -> Q/1
  RST/1 -> Register/2

== system volo_agcdc_pipelined/TOP_LEVEL_AGC_TIMING/rising edge ==
  note: rising edge
  A : Inport
  Delay1 : xbsIndex_r4/Delay  rst=off  infoeditControl=Selection of Reset will increase slice count due to use of real FFs and instead of SRLs  en=off  latency=1  dbl_ovrd=off  reg_retiming=off  block_type=delay
  Inverter2 : xbsIndex_r4/Inverter  en=off  latency=0  dbl_ovrd=off  block_type=inv
  Logical2 : xbsIndex_r4/Logical  logical_function=AND  inputs=2  en=off  latency=0  precision=Full  arith_type=Unsigned  n_bits=16  bin_pt=0  align_bp=on  dbl_ovrd=off  block_type=logical
  Q : Outport
  wires:
  Logical2/1 -> Q/1
  A/1 -> Logical2/1, Delay1/1
  Delay1/1 -> Inverter2/1
  Inverter2/1 -> Logical2/2

== system volo_agcdc_pipelined/AGC_SETGAIN_CONTROLLER/SPI_Controller1/Hold For 8 ==
  A : Inport
  Constant : xbsIndex_r4/Constant  const=7  gui_display_data_type=Fixed-point  arith_type=Unsigned  n_bits=8  bin_pt=0  preci_type=Single  exp_width=8  frac_width=24  explicit_period=off  period=1  equ=P=C  opselect=C  inp2=PCIN>>17  opr=+  inp1=P  carry=CIN  dbl_ovrd=off  block_type=constant
  Counter : xbsIndex_r4/Counter  cnt_type=Free Running  cnt_to=Inf  operation=Up  start_count=0  cnt_by_val=1  arith_type=Unsigned  n_bits=8  bin_pt=0  load_pin=off  rst=on  en=on  explicit_period=on  period=1  dbl_ovrd=off  use_behavioral_HDL=off  implementation=Fabric  block_type=counter
  Inverter : xbsIndex_r4/Inverter  en=off  latency=0  dbl_ovrd=off  block_type=inv
  Logical : xbsIndex_r4/Logical  logical_function=OR  inputs=2  en=off  latency=0  precision=Full  arith_type=Unsigned  n_bits=16  bin_pt=0  align_bp=on  dbl_ovrd=off  block_type=logical
  Relational : xbsIndex_r4/Relational  mode=a=b  en=off  latency=0  dbl_ovrd=off  block_type=relational
  rising edge3 : Subsystem
  Q : Outport
  wires:
  rising edge3/1(Q) -> Counter/1, Logical/1  "init_pulse"
  A/1 -> rising edge3/1(A)
  Logical/1 -> Q/1
  Inverter/1 -> Logical/2, Counter/2  "timer_counting"
  Constant/1 -> Relational/1
  Counter/1 -> Relational/2
  Relational/1 -> Inverter/1

== system volo_agcdc_pipelined/AGC_SETGAIN_CONTROLLER/SPI_Controller1/SPITimeout OneShot ==
  Start : Inport
  CountTo : Inport  Port=2
  RST : Inport  Port=3
  HoldUntilReset : Subsystem
  Inverter2 : xbsIndex_r4/Inverter  en=off  latency=0  dbl_ovrd=off  block_type=inv
  Logical5 : xbsIndex_r4/Logical  logical_function=AND  inputs=2  en=off  latency=0  precision=Full  arith_type=Unsigned  n_bits=16  bin_pt=0  align_bp=on  dbl_ovrd=off  block_type=logical
  PayloadTimeoutCounter : xbsIndex_r4/Counter  cnt_type=Free Running  cnt_to=Inf  operation=Up  start_count=0  cnt_by_val=1  arith_type=Unsigned  n_bits=12  bin_pt=0  load_pin=off  rst=on  en=on  explicit_period=on  period=1  dbl_ovrd=off  use_behavioral_HDL=off  implementation=Fabric  block_type=counter
  Relational2 : xbsIndex_r4/Relational  mode=a=b  en=off  latency=0  dbl_ovrd=off  block_type=relational
  Done : Outport
  wires:
  RST/1 -> HoldUntilReset/2(RST), PayloadTimeoutCounter/1
  CountTo/1 -> Relational2/2
  PayloadTimeoutCounter/1 -> Relational2/1
  Relational2/1 -> Inverter2/1, Done/1  "payloadTimeout"
  Inverter2/1 -> Logical5/2
  Logical5/1 -> PayloadTimeoutCounter/2
  Start/1 -> HoldUntilReset/1(A)
  HoldUntilReset/1(Q) -> Logical5/1

== system volo_agcdc_pipelined/AGC_SETGAIN_CONTROLLER/SPI_Controller1/SR-Latch ==
  S : Inport
  R : Inport  Port=2
  Register : xbsIndex_r4/Register  init=0  rst=on  en=on  dbl_ovrd=off  block_type=register
  Q : Outport
  wires:
  S/1 -> Register/3, Register/1
  Register/1 -> Q/1
  R/1 -> Register/2

== system volo_agcdc_pipelined/AGC_SETGAIN_CONTROLLER/SPI_Controller1/SR-Latch1 ==
  S : Inport
  R : Inport  Port=2
  Register : xbsIndex_r4/Register  init=0  rst=on  en=on  dbl_ovrd=off  block_type=register
  Q : Outport
  wires:
  S/1 -> Register/3, Register/1
  Register/1 -> Q/1
  R/1 -> Register/2

== system volo_agcdc_pipelined/AGC_SETGAIN_CONTROLLER/SPI_Controller1/Write Pulse Buffer ==
  SPIBusy : Inport
  Write : Inport  Port=2
  Inverter2 : xbsIndex_r4/Inverter  en=off  latency=0  dbl_ovrd=off  block_type=inv
  Logical1 : xbsIndex_r4/Logical  logical_function=AND  inputs=2  en=off  latency=0  precision=Full  arith_type=Unsigned  n_bits=16  bin_pt=0  align_bp=on  dbl_ovrd=off  block_type=logical
  Logical2 : xbsIndex_r4/Logical  logical_function=AND  inputs=2  en=off  latency=0  precision=Full  arith_type=Unsigned  n_bits=16  bin_pt=0  align_bp=on  dbl_ovrd=off  block_type=logical
  Logical3 : xbsIndex_r4/Logical  logical_function=OR  inputs=2  en=off  latency=0  precision=Full  arith_type=Unsigned  n_bits=16  bin_pt=0  align_bp=on  dbl_ovrd=off  block_type=logical
  Logical4 : xbsIndex_r4/Logical  logical_function=AND  inputs=2  en=off  latency=0  precision=Full  arith_type=Unsigned  n_bits=16  bin_pt=0  align_bp=on  dbl_ovrd=off  block_type=logical
  SR-Latch : Subsystem
  Start : Outport
  wires:
  Logical3/1 -> Start/1, SR-Latch/2(R)  "Reset Pulse Buffer"
  Logical2/1 -> SR-Latch/1(S)  "Buffer Write Pulse"
  SPIBusy/1 -> Logical2/1, Inverter2/1  "SPI Busy"
  Logical4/1 -> Logical3/2  "Passthrough Write Pulse"
  Write/1 -> Logical4/1, Logical2/2  "Write Pulse"
  Inverter2/1 -> Logical1/2, Logical4/2  "SPI Idle"
  SR-Latch/1(Q) -> Logical1/1  "Buffered Pulse Waiting"
  Logical1/1 -> Logical3/1  "Buffered Pulse"

== system volo_agcdc_pipelined/AGC_SETGAIN_CONTROLLER/SPI_Controller1/rising edge ==
  note: rising edge
  A : Inport
  Delay1 : xbsIndex_r4/Delay  rst=off  infoeditControl=Selection of Reset will increase slice count due to use of real FFs and instead of SRLs  en=off  latency=1  dbl_ovrd=off  reg_retiming=off  block_type=delay
  Inverter2 : xbsIndex_r4/Inverter  en=off  latency=0  dbl_ovrd=off  block_type=inv
  Logical2 : xbsIndex_r4/Logical  logical_function=AND  inputs=2  en=off  latency=0  precision=Full  arith_type=Unsigned  n_bits=16  bin_pt=0  align_bp=on  dbl_ovrd=off  block_type=logical
  Q : Outport
  wires:
  Logical2/1 -> Q/1
  A/1 -> Logical2/1, Delay1/1
  Delay1/1 -> Inverter2/1
  Inverter2/1 -> Logical2/2

== system volo_agcdc_pipelined/AGC_SETGAIN_CONTROLLER/SPI_Controller1/rising edge1 ==
  note: rising edge
  A : Inport
  Delay1 : xbsIndex_r4/Delay  rst=off  infoeditControl=Selection of Reset will increase slice count due to use of real FFs and instead of SRLs  en=off  latency=1  dbl_ovrd=off  reg_retiming=off  block_type=delay
  Inverter2 : xbsIndex_r4/Inverter  en=off  latency=0  dbl_ovrd=off  block_type=inv
  Logical2 : xbsIndex_r4/Logical  logical_function=AND  inputs=2  en=off  latency=0  precision=Full  arith_type=Unsigned  n_bits=16  bin_pt=0  align_bp=on  dbl_ovrd=off  block_type=logical
  Q : Outport
  wires:
  Inverter2/1 -> Logical2/2
  Delay1/1 -> Inverter2/1
  A/1 -> Delay1/1, Logical2/1
  Logical2/1 -> Q/1

== system volo_agcdc_pipelined/AGC_SETGAIN_CONTROLLER/SPI_Controller1/rising edge2 ==
  note: rising edge
  A : Inport
  Delay1 : xbsIndex_r4/Delay  rst=off  infoeditControl=Selection of Reset will increase slice count due to use of real FFs and instead of SRLs  en=off  latency=1  dbl_ovrd=off  reg_retiming=off  block_type=delay
  Inverter2 : xbsIndex_r4/Inverter  en=off  latency=0  dbl_ovrd=off  block_type=inv
  Logical2 : xbsIndex_r4/Logical  logical_function=AND  inputs=2  en=off  latency=0  precision=Full  arith_type=Unsigned  n_bits=16  bin_pt=0  align_bp=on  dbl_ovrd=off  block_type=logical
  Q : Outport
  wires:
  Logical2/1 -> Q/1
  A/1 -> Logical2/1, Delay1/1
  Delay1/1 -> Inverter2/1
  Inverter2/1 -> Logical2/2
